simulink model "gravity"  (R2015a)
settings: Solver=ode23s  StartTime=0.0  StopTime=100000  RelTol=1e-3
libraries: simulink x1
settings Model: Creator=moritz  LastModifiedBy=moritz
settings SolverCC: ShapePreserveControl=EnableAll

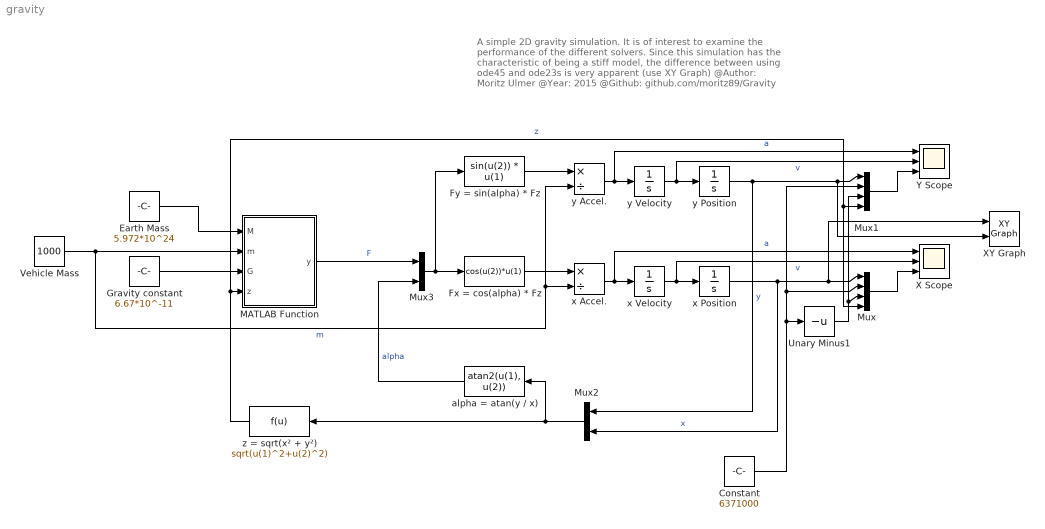
== system gravity ==
  note: A simple 2D gravity simulation. It is of interest to examine the
      | performance of the different solvers. Since this simulation has
      | the characteristic of being a stiff model, the difference between
      | using ode45 and ode23s is very apparent (use XY Graph)
      | @Author: Moritz Ulmer
      | @Year: 2015
      | @Github: github.com/moritz89/Gravity
  Constant : Constant  Value=6371000
  Earth Mass : Constant  Value=5.972*10^24
  Fx = cos(alpha) * Fz : Fcn  Expr=cos(u(2))*u(1)
  Fy = sin(alpha) * Fz : Fcn  Expr=sin(u(2)) * u(1)
  Gravity constant : Constant  Value=6.67*10^-11
  MATLAB Function : MATLAB Function  TreatAsAtomicUnit=on
  Mux : Mux
  Mux1 : Mux
  Mux2 : Mux  Inputs=2
  Mux3 : Mux  Inputs=2
  Unary Minus1 : UnaryMinus
  Vehicle Mass : Constant  Value=1000
  X Scope : Scope  NumInputPorts=3
      settings: TimeRange=100000  YMin=-5~-5~-5  YMax=5~5~5
  XY Graph : simulink/Sinks/XY Graph  xmin=-20000000  xmax=20000000  ymin=-20000000  ymax=20000000  st=-1
  Y Scope : Scope  NumInputPorts=3
      settings: YMin=-5~-5~-5  YMax=5~5~5
  alpha = atan(y / x) : Fcn  Expr=atan2(u(1), u(2))
  x Accel. : Product  Inputs=*/
  x Position : Integrator  InitialCondition=6371000+7000000
  x Velocity : Integrator
  y Accel. : Product  Inputs=*/
  y Position : Integrator
  y Velocity : Integrator  InitialCondition=5000
  z = sqrt(x² + y²) : Fcn  Expr=sqrt(u(1)^2+u(2)^2)
  wires:
  Vehicle Mass/1 -> y Accel./2, x Accel./2, MATLAB Function/2(m)  "m"
  Gravity constant/1 -> MATLAB Function/3(G)
  x Position/1 -> Mux2/2, XY Graph/1, Mux/1  "x"
  Earth Mass/1 -> MATLAB Function/1(M)
  MATLAB Function/1(y) -> Mux3/1  "F"
  x Accel./1 -> X Scope/1, x Velocity/1  "a"
  x Velocity/1 -> X Scope/2, x Position/1  "v"
  Mux/1 -> X Scope/3
  Constant/1 -> Unary Minus1/1, Mux1/2, Mux/2
  Unary Minus1/1 -> Mux1/3, Mux/3
  y Accel./1 -> Y Scope/1, y Velocity/1  "a"
  y Velocity/1 -> Y Scope/2, y Position/1  "v"
  y Position/1 -> Mux2/1, Mux1/1, XY Graph/2  "y"
  Mux1/1 -> Y Scope/3
  Mux2/1 -> alpha = atan(y / x)/1, z = sqrt(x² + y²)/1
  z = sqrt(x² + y²)/1 -> Mux1/4, Mux/4, MATLAB Function/4(z)  "z"
  Fx = cos(alpha) * Fz/1 -> x Accel./1
  Fy = sin(alpha) * Fz/1 -> y Accel./1
  alpha = atan(y / x)/1 -> Mux3/2  "alpha"
  Mux3/1 -> Fy = sin(alpha) * Fz/1, Fx = cos(alpha) * Fz/1

== matlab function gravity/MATLAB Function ==
  data: M input; y output; m input; G input; z input
function y = fcn(M, m, G, z)
%#codegen

    y = G*M*m/(z^2)*sign(-z);
